simulink model "AsynchronousMotionPlanner"  (R2025b)
settings: Solver=FixedStepAuto  StartTime=0.0  StopTime=50  FixedStep=0.1  RelTol=1e-3  EnableMultiTasking=on
undefined symbols (not defined in the file): structMotionPlannerIn
libraries: AVE_Library x2, MotionPlanner_Library x1
settings Model: Creator=damerius  LastModifiedBy=Scythe
settings SolverCC: ConcurrentTasks=on
settings DataIOCC: SaveOutput=off  SignalLogging=off  DSMLogging=off  SaveTime=off  ReturnWorkspaceOutputs=off
settings OptimizationCC: DefaultParameterBehavior=Inlined  ZeroExternalMemoryAtStartup=off  ZeroInternalMemoryAtStartup=off  SimCompilerOptimization=on
settings DebuggingCC: UnconnectedInputMsg=warning  UnconnectedOutputMsg=warning  UnconnectedLineMsg=warning
settings HardwareCC: ProdBitPerLong=64.0  ProdHWDeviceType=Intel->x86-64 (Linux 64)  TargetBitPerLong=64.0  TargetBitPerPointer=64.0  TargetBitPerSizeT=64.0  TargetBitPerPtrDiffT=64.0  TargetLargestAtomicFloat=Float  TargetIntDivRoundTo=Zero  TargetEndianess=LittleEndian  TargetWordSize=64.0  TargetHWDeviceType=Intel->x86-64 (Linux 64)  ProdEqTarget=off
settings ModelReferenceCC: EnableRefExpFcnMdlSchedulingChecks=on
settings SFSimCC: SimParseCustomCode=off  SimGenImportedTypeDefs=on  SimTargetLang=C++  SimDLTargetLibrary=mkl-dnn
settings RTWCC: GenCodeOnly=on  PackageGeneratedCodeAndArtifacts=on  PackageName=PackNGo  BuildConfiguration=Faster Runs  TargetLang=C++
settings CodeAppCC: ForceParamTrailComments=on  MaxIdLength=128.0  StateflowObjectComments=on  MATLABSourceComments=on  UseSimReservedNames=on
settings GRTTargetCC: TargetLangStandard=C++20 (ISO)  MatFileLogging=off  CodeInterfacePackaging=C++ class  SubcomponentCodeInterfacePackaging=C++ class

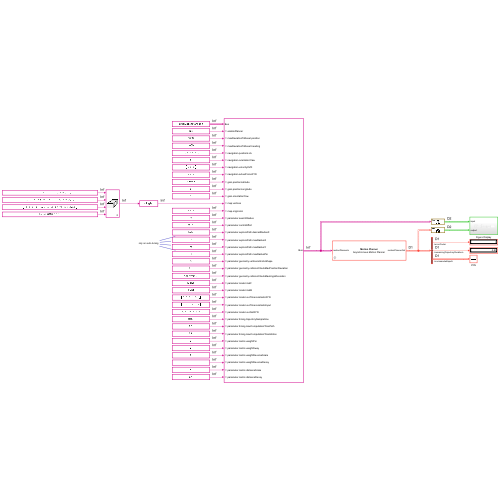
[thumbnail: Simulink's stored preview of the top-level diagram]
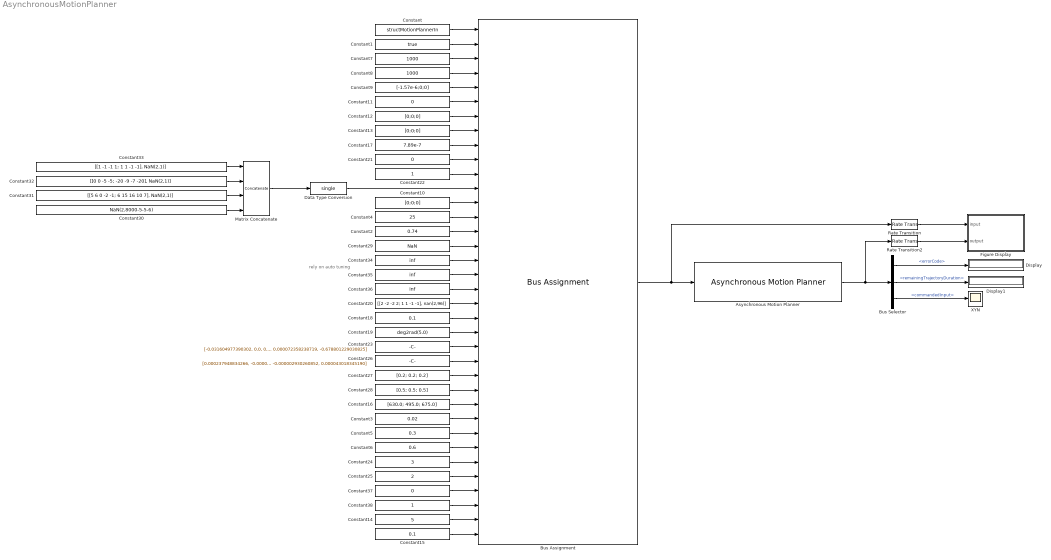
== system AsynchronousMotionPlanner ==
  note: rely on auto tuning
  Asynchronous Motion Planner : MotionPlanner_Library/Asynchronous Motion Planner  priorityWorkerThread=40  mpsvCPUCoresToUse=int32(0:7)  sampletime=0.1
  Bus Assignment : BusAssignment  AssignedSignals=enablePlanner,maxDeviationToReset.position,maxDeviationToReset.heading,navigation.positionLLA,navigation.orientationYaw,navigation.velocityUVR,navigation.actualForceXYN,goal.positionLatitude,goal.positionLongitude,goal.orientationYaw,map.vertices,map.originLLA,parameter.searchRadius,parameter.controlEffort,parameter.explorePath.desiredRadiusX,parameter.explorePath.maxRadiusX,parameter.explorePath.maxRadiusY,parameter.explorePath.maxRadiusPsi,parameter.geometry.verticesVehicleShape,parameter.geometry.collisionCheckMaxPositionDeviation,parameter.geometry.collisionCheckMaxAngleDeviation,parameter.model.matF,parameter.model.matB,parameter.model.vecTimeconstantsXYN,parameter.model.vecTimeconstantsInput,parameter.model.vecSatXYN,parameter.timing.trajectorySampletime,parameter.timing.maxComputationTimePath,parameter.timing.maxComputationTimeMotion,parameter.metric.weightPsi,parameter.metric.weightSway,parameter.metric.weightReverseScale,parameter.metric.weightReverseDecay,parameter.metric.distanceScale,parameter.metric.distanceDecay
  Bus Selector : BusSelector  OutputSignals=errorCode,controlCommand.remainingTrajectoryDuration,controlCommand.commandedInput
  Constant : Constant  Value=structMotionPlannerIn  OutDataTypeStr=Bus: busMotionPlannerIn  SampleTime=Inf
  Constant1 : Constant  Value=true
  Constant10 : Constant  Value=[0;0;0]  OutDataTypeStr=double
  Constant11 : Constant  Value=0  OutDataTypeStr=double
  Constant12 : Constant  Value=[0;0;0]  OutDataTypeStr=double
  Constant13 : Constant  Value=[0;0;0]  OutDataTypeStr=double
  Constant14 : Constant  Value=5  OutDataTypeStr=double
  Constant15 : Constant  Value=0.1  OutDataTypeStr=double
  Constant16 : Constant  Value=[630.0; 495.0; 675.0]  OutDataTypeStr=double
  Constant17 : Constant  Value=7.89e-7  OutDataTypeStr=double
  Constant18 : Constant  Value=0.1  OutDataTypeStr=double
  Constant19 : Constant  Value=deg2rad(5.0)  OutDataTypeStr=double
  Constant2 : Constant  Value=0.74  OutDataTypeStr=double
  Constant20 : Constant  Value=[[2 -2 -2 2; 1 1 -1 -1], nan(2,96)]  OutDataTypeStr=single
  Constant21 : Constant  Value=0  OutDataTypeStr=double
  Constant22 : Constant  OutDataTypeStr=double
  Constant23 : Constant  Value=[-0.031604977390302, 0.0, 0.0, 0.233741474945168, 0.0, 0.0, 0.0, 0.0, 0.133462292221887, -0.020792892088185, 0.0, 0.0; 0.0, -0.041708610292712, 0.017242263124379, 0.0, -0.251243228165994, -0.000476044356140, 0.0, 0.0, 0.005297185500344, 0.0, -0.167981638498434, 0.497442136687157; 0.0, 0.000017966020615, -0.023528504195578, 0.0, 0.000108223241795, 0.000649602175186, 0.0, 0.0, -0.000002281767319, 0.0, 0.000072358238719, -0.678801229030825]  OutDataTypeStr=double
  Constant24 : Constant  Value=3  OutDataTypeStr=double
  Constant25 : Constant  Value=2  OutDataTypeStr=double
  Constant26 : Constant  Value=[0.000237948834266, -0.000004551592718, 0.000010003488944; -0.000009313932115, 0.000215194147058, -0.000024957572224; -0.000002202124158, -0.000002930260852, 0.000043018345190]  OutDataTypeStr=double
  Constant27 : Constant  Value=[0.2; 0.2; 0.2]  OutDataTypeStr=double
  Constant28 : Constant  Value=[0.5; 0.5; 0.5]  OutDataTypeStr=double
  Constant29 : Constant  Value=NaN  OutDataTypeStr=double
  Constant3 : Constant  Value=0.02  OutDataTypeStr=double
  Constant30 : Constant  Value=NaN(2,8000-5-5-6)
  Constant31 : Constant  Value=[[5 6 0 -2 -1; 6 15 16 10 7], NaN(2,1)]
  Constant32 : Constant  Value=[[0 0 -5 -5; -20 -9 -7 -20], NaN(2,1)]
  Constant33 : Constant  Value=[[1 -1 -1 1; 1 1 -1 -1], NaN(2,1)]
  Constant34 : Constant  Value=inf  OutDataTypeStr=double
  Constant35 : Constant  Value=inf  OutDataTypeStr=double
  Constant36 : Constant  Value=inf  OutDataTypeStr=double
  Constant37 : Constant  Value=0  OutDataTypeStr=double
  Constant38 : Constant  OutDataTypeStr=double
  Constant4 : Constant  Value=25  OutDataTypeStr=double
  Constant5 : Constant  Value=0.3  OutDataTypeStr=double
  Constant6 : Constant  Value=0.6  OutDataTypeStr=double
  Constant7 : Constant  Value=1000  OutDataTypeStr=double
  Constant8 : Constant  Value=1000  OutDataTypeStr=double
  Constant9 : Constant  Value=[-1.57e-6;0;0]  OutDataTypeStr=double
  Data Type Conversion : DataTypeConversion  OutDataTypeStr=single  SaturateOnIntegerOverflow=off  RndMeth=Floor
  Display : Display
  Display1 : Display
  Figure Display : Subsystem
  Matrix Concatenate : Concatenate  NumInputs=4  Mode=Multidimensional array  ConcatenateDimension=2
  Rate Transition : RateTransition  Deterministic=off  OutPortSampleTime=1
  Rate Transition2 : RateTransition  Deterministic=off  OutPortSampleTime=1
  XYN : Scope
      settings: ActiveDisplayYMinimum=-805.40887957488792  ActiveDisplayYMaximum=789.48574320118462
  wires:
  Constant/1 -> Bus Assignment/1
  Bus Assignment/1 -> Asynchronous Motion Planner/1, Rate Transition/1
  Constant1/1 -> Bus Assignment/2
  Constant20/1 -> Bus Assignment/20
  Constant2/1 -> Bus Assignment/15
  Constant18/1 -> Bus Assignment/21
  Constant19/1 -> Bus Assignment/22
  Constant23/1 -> Bus Assignment/23
  Constant26/1 -> Bus Assignment/24
  Constant28/1 -> Bus Assignment/26
  Constant27/1 -> Bus Assignment/25
  Constant16/1 -> Bus Assignment/27
  Constant3/1 -> Bus Assignment/28
  Constant5/1 -> Bus Assignment/29
  Constant6/1 -> Bus Assignment/30
  Constant24/1 -> Bus Assignment/31
  Constant25/1 -> Bus Assignment/32
  Constant37/1 -> Bus Assignment/33
  Constant38/1 -> Bus Assignment/34
  Constant15/1 -> Bus Assignment/36
  Constant14/1 -> Bus Assignment/35
  Constant4/1 -> Bus Assignment/14
  Constant7/1 -> Bus Assignment/3
  Constant8/1 -> Bus Assignment/4
  Constant9/1 -> Bus Assignment/5
  Constant10/1 -> Bus Assignment/13
  Constant11/1 -> Bus Assignment/6
  Constant12/1 -> Bus Assignment/7
  Constant13/1 -> Bus Assignment/8
  Constant17/1 -> Bus Assignment/9
  Constant21/1 -> Bus Assignment/10
  Constant22/1 -> Bus Assignment/11
  Data Type Conversion/1 -> Bus Assignment/12
  Asynchronous Motion Planner/1 -> Rate Transition2/1, Bus Selector/1
  Bus Selector/1 -> Display/1  "<errorCode>"
  Bus Selector/2 -> Display1/1  "<remainingTrajectoryDuration>"
  Bus Selector/3 -> XYN/1  "<commandedInput>"
  Matrix Concatenate/1 -> Data Type Conversion/1
  Constant32/1 -> Matrix Concatenate/2
  Constant31/1 -> Matrix Concatenate/3
  Constant30/1 -> Matrix Concatenate/4
  Constant33/1 -> Matrix Concatenate/1
  Rate Transition2/1 -> Figure Display/2(output)
  Rate Transition/1 -> Figure Display/1(input)
  Constant29/1 -> Bus Assignment/16
  Constant34/1 -> Bus Assignment/17
  Constant35/1 -> Bus Assignment/18
  Constant36/1 -> Bus Assignment/19

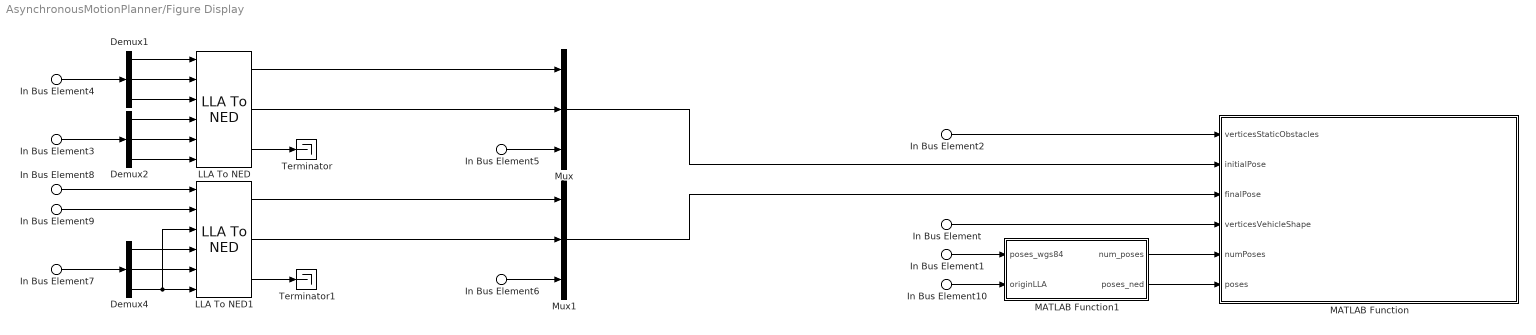
== system AsynchronousMotionPlanner/Figure Display ==
  In Bus Element : Inport  PortName=input  Element=parameter.geometry.verticesVehicleShape
  In Bus Element2 : Inport  PortName=input  Element=map.vertices
  In Bus Element3 : Inport  PortName=input  Element=map.originLLA
  In Bus Element7 : Inport  PortName=input  Element=map.originLLA
  In Bus Element10 : Inport  PortName=input  Element=map.originLLA
  In Bus Element4 : Inport  PortName=input  Element=navigation.positionLLA
  In Bus Element5 : Inport  PortName=input  Element=navigation.orientationYaw
  In Bus Element6 : Inport  PortName=input  Element=goal.orientationYaw
  In Bus Element8 : Inport  PortName=input  Element=goal.positionLatitude
  In Bus Element9 : Inport  PortName=input  Element=goal.positionLongitude
  In Bus Element1 : Inport  Port=2  PortName=output  Element=path.poses
  Demux1 : Demux  Outputs=3
  Demux2 : Demux  Outputs=3
  Demux4 : Demux  Outputs=3
  LLA To NED : AVE_Library/Essential/Transformation/LLA To NED
      settings: SourceProductName=AVE - Autonomous Vehicle Control Toolbox
  LLA To NED1 : AVE_Library/Essential/Transformation/LLA To NED
      settings: SourceProductName=AVE - Autonomous Vehicle Control Toolbox
  MATLAB Function : MATLAB Function  TreatAsAtomicUnit=on
  MATLAB Function1 : MATLAB Function  TreatAsAtomicUnit=on
  Mux : Mux  Inputs=3
  Mux1 : Mux  Inputs=3
  Terminator : Terminator
  Terminator1 : Terminator
  wires:
  In Bus Element4/1 -> Demux1/1
  Demux1/1 -> LLA To NED/1
  Demux1/2 -> LLA To NED/2
  Demux1/3 -> LLA To NED/3
  In Bus Element3/1 -> Demux2/1
  Demux2/1 -> LLA To NED/4
  Demux2/2 -> LLA To NED/5
  Demux2/3 -> LLA To NED/6
  LLA To NED/3 -> Terminator/1
  LLA To NED/1 -> Mux/1
  LLA To NED/2 -> Mux/2
  In Bus Element5/1 -> Mux/3
  In Bus Element/1 -> MATLAB Function/4(verticesVehicleShape)
  In Bus Element2/1 -> MATLAB Function/1(verticesStaticObstacles)
  Mux/1 -> MATLAB Function/2(initialPose)
  Mux1/1 -> MATLAB Function/3(finalPose)
  In Bus Element6/1 -> Mux1/3
  Demux4/3 -> LLA To NED1/3, LLA To NED1/6
  Demux4/2 -> LLA To NED1/5
  Demux4/1 -> LLA To NED1/4
  In Bus Element7/1 -> Demux4/1
  LLA To NED1/1 -> Mux1/1
  LLA To NED1/2 -> Mux1/2
  In Bus Element8/1 -> LLA To NED1/1
  In Bus Element9/1 -> LLA To NED1/2
  LLA To NED1/3 -> Terminator1/1
  In Bus Element1/1 -> MATLAB Function1/1(poses_wgs84)
  MATLAB Function1/1(num_poses) -> MATLAB Function/5(numPoses)
  MATLAB Function1/2(poses_ned) -> MATLAB Function/6(poses)
  In Bus Element10/1 -> MATLAB Function1/2(originLLA)

== matlab function AsynchronousMotionPlanner/Figure Display/MATLAB Function1 ==
  data: poses_wgs84 input; num_poses output; originLLA input; poses_ned output
function [num_poses, poses_ned] = fcn(poses_wgs84, originLLA)
    num_poses = 0;
    poses_ned = poses_wgs84;
    for i = 1:size(poses_wgs84,2)
        if(~isfinite(poses_wgs84(1,i)) || ~isfinite(poses_wgs84(2,i)) || ~isfinite(poses_wgs84(3,i)))
            break;
        end
        num_poses = num_poses + 1;
        [N, E, ~] = ave.LLA2NED(poses_wgs84(1,i), poses_wgs84(2,i), originLLA(3), originLLA(1), originLLA(2), originLLA(3));
        poses_ned(:,i) = [N; E; poses_wgs84(3,i)];
    end
end

== matlab function AsynchronousMotionPlanner/Figure Display/MATLAB Function ==
  data: verticesStaticObstacles input; initialPose input; finalPose input; verticesVehicleShape input; numPoses input; poses input
function FigureDisplay(verticesStaticObstacles, initialPose, finalPose, verticesVehicleShape, numPoses, poses)
    persistent f;
    if(isempty(f))
        f = figure(42);
    end

    clf;
    hold on;
    PlotPath(numPoses, poses, verticesVehicleShape, [0 0.3 0.5]);
    PlotVehicleShape(initialPose, verticesVehicleShape, [0.9 0 0]);
    PlotVehicleShape(finalPose, verticesVehicleShape, [0 0.7 0]);
    PlotObstacles(verticesStaticObstacles);
    view(90,-90);
    axis equal;
    box on;
    grid on;
    xlabel('x in m');
    ylabel('y in m');
    drawnow();
end

function PlotPath(numPoses, poses, verticesVehicleShape, color)
    x = poses(1,1:numPoses);
    y = poses(2,1:numPoses);
    plot(x,y,'LineWidth',2,'Color',color);
    for i = uint32(1):uint32(numPoses)
        PlotVehicleShape(poses(:,i), verticesVehicleShape, color);
    end
end

function PlotVehicleShape(pose, verticesVehicleShape, color)
    c = cos(pose(3));
    s = sin(pose(3));
    R = [c -s; s c];

    N = int32(size(verticesVehicleShape,2));
    i0 = int32(-1);

    for i = int32(1):N
        finiteVertex = isfinite(verticesVehicleShape(1,i)) && isfinite(verticesVehicleShape(2,i));
        if((i0 < 1) && finiteVertex)
            i0 = i;
        elseif((i0 > 0) && (~finiteVertex || (i == N)))
            i = i + int32((i == N) && finiteVertex);
            vertices = R * verticesVehicleShape(:,i0:(i-1)) + [pose(1); pose(2)];
            PlotPolygon(vertices, color);
            plot(pose(1),pose(2),'o','Color',color);
            i0 = int32(-1);
        end
    end
end

function PlotObstacles(verticesStaticObstacles)
    N = int32(size(verticesStaticObstacles,2));
    i0 = int32(-1);

    for i = int32(1):N
        finiteVertex = isfinite(verticesStaticObstacles(1,i)) && isfinite(verticesStaticObstacles(2,i));
        if((i0 < 1) && finiteVertex)
            i0 = i;
        elseif((i0 > 0) && (~finiteVertex || (i == N)))
            i = i + int32((i == N) && finiteVertex);
            PlotPolygon(verticesStaticObstacles(:,i0:(i-1)), [0,0,0]);
            i0 = int32(-1);
        end
    end
end

function PlotPolygon(vertices, color)
    x = [vertices(1,:) vertices(1,1)];
    y = [vertices(2,:) vertices(2,1)];
    plot(x,y,'LineWidth',1,'Color',color);
end
